simulink model "AttitudeComplementary2"  (Simulink 6.6)
settings: Solver=ode4  StartTime=0.0  StopTime=80  FixedStep=SampleT  RelTol=1e-3
InitFcn:
  | clc
  | Taxi_Var_new
  | failures
  | insInit
  | piccolo_init
values from neighbouring files (symbols this model uses):
  A1 = 0    [Taxi_Var.m]    (also in Taxi_Var_new.m = 0.007)
  Apolar = 0.0899    [Taxi_Var.m]    (also in Taxi_Var_new.m = 0.057)
  APtsamp = 0.005    [failures.m]    (also in piccolo_init.m = 0.05)
  CD0 = 0.0219    [Taxi_Var.m]    (also in Taxi_Var_new.m = 0.022)
  chord = S/span    (= 0.384036716878)    [Taxi_Var.m]    (also in Taxi_Var_new.m = 0.351341681574)
  CL0 = 0.1857    [Taxi_Var.m]    (also in Taxi_Var_new.m = 0.38)
  CLa = 4.6206    [Taxi_Var.m]    (also in Taxi_Var_new.m = 18.5)
  CLa_dot = 1.93    [Taxi_Var.m]    (also in Taxi_Var_new.m = 2.64)
  Clb = -0.0043    [Taxi_Var.m]    (also in Taxi_Var_new.m = -0.06)
  ClDa = 0.1695    [Taxi_Var.m]    (also in Taxi_Var_new.m)
  CLDe = 0.4032    [Taxi_Var.m]    (also in Taxi_Var_new.m = 0.24)
  CLDf = 0.047    [Taxi_Var.m]    (also in Taxi_Var_new.m = 0.4)
  ClDr = 0.0003    [Taxi_Var.m]    (also in Taxi_Var_new.m = 0.055)
  Clp = -0.4425    [Taxi_Var.m]    (also in Taxi_Var_new.m = -0.88)
  CLq = 8.7465    [Taxi_Var.m]    (also in Taxi_Var_new.m = 7.4)
  Clr = 0.0675    [Taxi_Var.m]    (also in Taxi_Var_new.m = 0.04)
  Cm0 = -0.0902    [Taxi_Var.m]    (also in Taxi_Var_new.m = 0.56)
  Cma = -1.3995    [Taxi_Var.m]    (also in Taxi_Var_new.m = -1.58)
  CmDe = -0.9493    [Taxi_Var.m]    (also in Taxi_Var_new.m = -41)
  CmDf = -.021    (= -0.021)    [Taxi_Var.m]    (also in Taxi_Var_new.m)
  Cmq = -10.8760    (= -10.876)    [Taxi_Var.m]    (also in Taxi_Var_new.m = -12)
  Cnb = 0.0281    [Taxi_Var.m]    (also in Taxi_Var_new.m = 0.73)
  CnDa = -0.0031    [Taxi_Var.m]    (also in Taxi_Var_new.m = -0.032)
  CnDr = -0.0882    [Taxi_Var.m]    (also in Taxi_Var_new.m = 0.19)
  Cnp = -0.0695    [Taxi_Var.m]    (also in Taxi_Var_new.m = -0.1)
  Cnr = -0.1045    [Taxi_Var.m]    (also in Taxi_Var_new.m = -0.23)
  CYb = -0.1999    [Taxi_Var.m]    (also in Taxi_Var_new.m = -0.98)
  CYDr = 0.0192    [Taxi_Var.m]    (also in Taxi_Var_new.m = 0.066)
  damax = 25*deg2rad    (= 0.436332312999)    [Taxi_Var.m]    (also in piccolo_init.m)
  damin = -25*deg2rad    (= -0.436332312999)    [Taxi_Var.m]    (also in piccolo_init.m)
  datrim = 0*deg2rad    (= 0)    [Taxi_Var.m]    (also in piccolo_init.m)
  demax = 15*deg2rad    (= 0.261799387799)    [Taxi_Var.m]    (also in piccolo_init.m)
  demin = -15*deg2rad    (= -0.261799387799)    [Taxi_Var.m]    (also in piccolo_init.m)
  detrim = -2.4137*deg2rad    (= -0.0421270121554)    [Taxi_Var.m]    (also in piccolo_init.m = -0.01308996939)
  dfland = 30*deg2rad    (= 0.523598775598)    [Taxi_Var.m]    (also in piccolo_init.m)
  dfmax = 30*deg2rad    (= 0.523598775598)    [Taxi_Var.m]    (also in piccolo_init.m)
  dfmin = 0*deg2rad    (= 0)    [Taxi_Var.m]    (also in piccolo_init.m)
  drmax = 25*deg2rad    (= 0.436332312999)    [Taxi_Var.m]    (also in piccolo_init.m)
  drmin = -25*deg2rad    (= -0.436332312999)    [Taxi_Var.m]    (also in piccolo_init.m)
  drtrim = 0*deg2rad    (= 0)    [Taxi_Var.m]    (also in piccolo_init.m)
  dtmax = 1    [Taxi_Var.m]    (also in piccolo_init.m)
  dtmin = 0    [Taxi_Var.m]    (also in piccolo_init.m)
  dttrim = 0.0725    [Taxi_Var.m]    (also in piccolo_init.m = 0.35)
  Euler_0 = [0; 0; 45]'*pi/180    [Taxi_Var.m]    (also in Taxi_Var_new.m = [0 0 45]'*pi/180)
  heightDown = 0    [insInit.m]
  heightUp = 3000    [insInit.m]
  IdxCmdOrbitRadius = 17    [piccolo_init.m]
  IdxCmdOrbitSense = 18    [piccolo_init.m]
  IdxCmdWp1Alt = 13    [piccolo_init.m]
  IdxCmdWp1Lat = 11    [piccolo_init.m]
  IdxCmdWp1Lon = 12    [piccolo_init.m]
  IdxCmdWp2Alt = 16    [piccolo_init.m]
  IdxCmdWp2Lat = 14    [piccolo_init.m]
  IdxCmdWp2Lon = 15    [piccolo_init.m]
  IdxEstimReserved1 = 4    [piccolo_init.m]
  IdxEstimWEast = 3    [piccolo_init.m]
  IdxEstimWNorth = 2    [piccolo_init.m]
  IdxGainsAltD = 10    [piccolo_init.m]
  IdxGainsAltI = 9    [piccolo_init.m]
  IdxGainsAltP = 8    [piccolo_init.m]
  IdxGainsPdynD = 4    [piccolo_init.m]
  IdxGainsPdynI = 3    [piccolo_init.m]
  IdxGainsPdynP = 2    [piccolo_init.m]
  IdxGainsPitchD = 7    [piccolo_init.m]
  IdxGainsPitchI = 6    [piccolo_init.m]
  IdxGainsPitchP = 5    [piccolo_init.m]
  IdxGainsRollD = 17    [piccolo_init.m]
  IdxGainsRollI = 16    [piccolo_init.m]
  IdxGainsRollP = 15    [piccolo_init.m]
  IdxGainsSlopeElevatorD = 25    [piccolo_init.m]
  IdxGainsSlopeElevatorP = 26    [piccolo_init.m]
  IdxGainsTrackConv = 24    [piccolo_init.m]
  IdxGainsTrackD = 23    [piccolo_init.m]
  IdxGainsTrackI = 22    [piccolo_init.m]
  IdxGainsTrackP = 21    [piccolo_init.m]
  IdxGainsTurnD = 14    [piccolo_init.m]
  IdxGainsTurnI = 13    [piccolo_init.m]
  IdxGainsTurnP = 12    [piccolo_init.m]
  IdxGainsYawD = 20    [piccolo_init.m]
  IdxGainsYawI = 19    [piccolo_init.m]
  IdxGainsYawP = 18    [piccolo_init.m]
  IdxLimitsAileronMax = 11    [piccolo_init.m]
  IdxLimitsAileronMin = 10    [piccolo_init.m]
  IdxLimitsBankMax = 9    [piccolo_init.m]
  IdxLimitsBankMin = 8    [piccolo_init.m]
  IdxLimitsElevatorMax = 13    [piccolo_init.m]
  IdxLimitsElevatorMin = 12    [piccolo_init.m]
  IdxLimitsFlapMax = 19    [piccolo_init.m]
  IdxLimitsFlapMin = 18    [piccolo_init.m]
  IdxLimitsPdynMax = 3    [piccolo_init.m]
  IdxLimitsPdynMin = 2    [piccolo_init.m]
  IdxLimitsRudderMax = 15    [piccolo_init.m]
  IdxLimitsRudderMin = 14    [piccolo_init.m]
  IdxLimitsThrottleMax = 17    [piccolo_init.m]
  IdxLimitsThrottleMin = 16    [piccolo_init.m]
  IdxSensorsAlt = 5    [piccolo_init.m]
  IdxSensorsLat = 3    [piccolo_init.m]
  IdxSensorsLon = 4    [piccolo_init.m]
  IdxSensorsVDown = 8    [piccolo_init.m]
  IdxSensorsVEast = 7    [piccolo_init.m]
  IdxSensorsVNorth = 6    [piccolo_init.m]
  IdxStatesGlobal = 2    [piccolo_init.m]
  IdxStatesManual = 16    [piccolo_init.m]
  IdxStatesMode = 15    [piccolo_init.m]
  ISA_g = 9.815    [Taxi_Var.m]    (also in Taxi_Var_new.m)
  ISA_hmax = 2000    [Taxi_Var.m]    (also in Taxi_Var_new.m)
  ISA_lapse = .0065    (= 0.0065)    [Taxi_Var.m]    (also in Taxi_Var_new.m)
  ISA_P0 = 101325    [Taxi_Var.m]    (also in Taxi_Var_new.m)
  ISA_R = 287    [Taxi_Var.m]    (also in Taxi_Var_new.m)
  ISA_rho0 = 1.225    [Taxi_Var.m]    (also in Taxi_Var_new.m)
  ISA_T0 = 289    [Taxi_Var.m]    (also in Taxi_Var_new.m)
  Ixx = 3.689084    [Taxi_Var.m]    (also in Taxi_Var_new.m = 3.8)
  Iyy = 7.43789    [Taxi_Var.m]    (also in Taxi_Var_new.m = 9.58)
  Izz = 10.22202    [Taxi_Var.m]    (also in Taxi_Var_new.m = 9.68)
  latDown = -100000    [insInit.m]
  latUp = 100000    [insInit.m]
  lonDown = -100000    [insInit.m]
  lonUp = 100000    [insInit.m]
  mass = 22.5    [Taxi_Var.m]    (also in Taxi_Var_new.m = 8.16466266)
  MinThK = 0.075    [Taxi_Var.m]    (also in Taxi_Var_new.m = 0.077)
  ... (+8 more)
undefined symbols (not defined in the file or in its folder): clock, DiscIntNeverNeededParam, Earth, gaind, polesd, WGS84, zerosd
libraries: piccolo_library x60, simulink x51, aerolibconvert2 x14, dspsigops x5, aerolibasang x5, aerolibatmos2 x2, aerolibtransform2 x2, aerolibnav x2, dspmtrx3 x1, aerolibutil x1
(part 2 of 6)

== system AttitudeComplementary2/Accel Comp/get Centripetal ==
  omega : Inport  Orientation=left
  Vb : Inport  Orientation=left  Port=2
  3vector LPF : Subsystem  Orientation=left  mask{flpf=0.1}
      mask prompts: flpf "LowPass Freq"
      mask Display: droots([],-flpf,flpf)
  3x3 Cross Product : aerolibutil/3x3 Cross Product  Orientation=left  SystemSampleTime=-1
  Integer Delay : simulink/Discrete/Integer Delay  Orientation=left  vinit=0.0  samptime=-1  NumDelays=1
  Integer Delay1 : simulink/Discrete/Integer Delay  Orientation=left  vinit=0.0  samptime=-1  NumDelays=1
  Saturation : Saturate  Orientation=left  UpperLimit=10  LowerLimit=-10
  w x Vb : Outport  Orientation=left
  wires:
  Integer Delay1/1 -> 3x3 Cross Product/1
  Integer Delay/1 -> 3x3 Cross Product/2
  omega/1 -> 3vector LPF/1(In1)
  Vb/1 -> Integer Delay/1
  3x3 Cross Product/1 -> Saturation/1  "w x Vb"
  3vector LPF/1(Out1) -> Integer Delay1/1
  Saturation/1 -> w x Vb/1

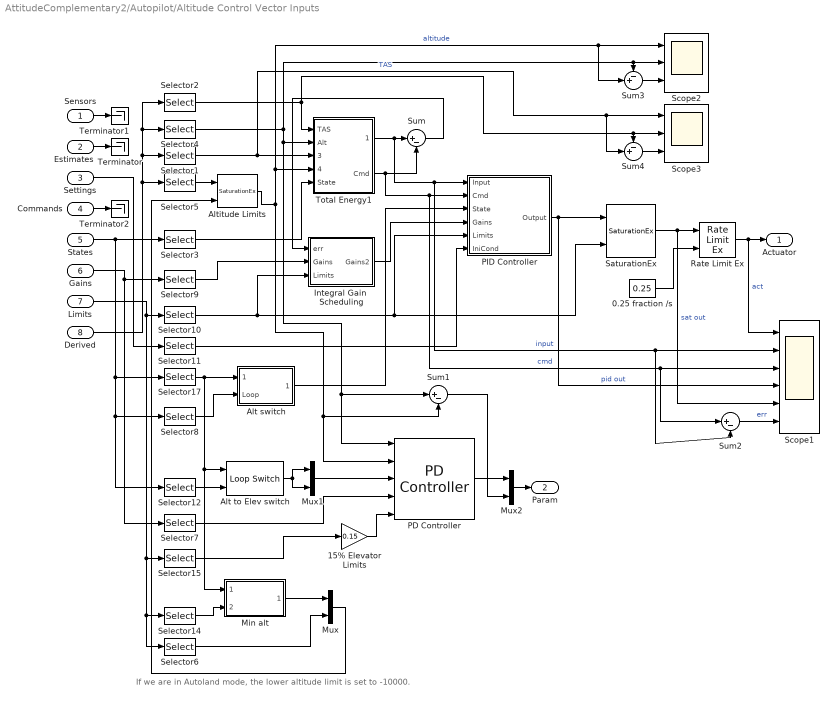
== system AttitudeComplementary2/Autopilot/Altitude Control Vector Inputs ==
  note: If we are in Autoland mode, the lower altitude limit is set to -10000.
  Sensors : Inport  PortDimensions=SizeSensors
  Estimates : Inport  Port=2  PortDimensions=SizeEstim
  Settings : Inport  Port=3  PortDimensions=SizeSet
  Commands : Inport  Port=4  PortDimensions=SizeCmd
  States : Inport  Port=5  PortDimensions=SizeStates
  Gains : Inport  Port=6  PortDimensions=SizeGains
  Limits : Inport  Port=7  PortDimensions=SizeLimits
  Derived : Inport  Port=8  PortDimensions=SizeDrv
  0.25 fraction /s : Constant  Value=0.25
  15% Elevator Limits : Gain  Gain=0.15  SaturateOnIntegerOverflow=on
  Alt switch : Subsystem  AncestorBlock=piccolo_library/Logic/DynP-Alt-Turn switch
  Alt to Elev switch : piccolo_library/Logic/Loop Switch  SystemSampleTime=-1
  Altitude Limits : piccolo_library/Nonlinear/SaturationEx  SystemSampleTime=-1
  Integral Gain  Scheduling : Subsystem
  Min alt : Subsystem
      mask Type: Loop Switch
      mask Description:
      | Select whether this individual loop is enabled or disabled.  This is done based on the specific
      | loop enable state, and the global flag.  In auto or manual steering the loop is on.  In Manual
      | or AutoLaunch the loop should be off.
  Mux : Mux  Inputs=2
  Mux1 : Mux  Inputs=2
  Mux2 : Mux  Inputs=2
  PD Controller : piccolo_library/Controllers/PD Controller  SystemSampleTime=-1  tsamp=tsamp  tdelay=0.5
  PID Controller : Subsystem  AncestorBlock=piccolo_library/Controllers/PID Controller  mask(PID Controller){tsamp=tsamp, tdelay=1}
      mask prompts: tsamp "Sample time:"; tdelay "Time derivative delay:"
      mask help: Generic PID (proportional, integral, derivative) controller with a single input and a single output.
  Rate Limit Ex : piccolo_library/Nonlinear/Rate Limit Ex  SystemSampleTime=-1  T=tsamp
  SaturationEx : piccolo_library/Nonlinear/SaturationEx  SystemSampleTime=-1
  Scope1 : Scope  NumInputPorts=6
      settings: YMin=0.120001~972.462~972.462~0.120001~0.120001~5.25e-006  YMax=0.120001~972.462~972.462~0.120001~0.120001~7e-006
  Scope2 : Scope  NumInputPorts=3
      settings: YMin=855~900.05~-0.475  YMax=945~900.475~-0.05  SaveName=ScopeData14
  Scope3 : Scope  NumInputPorts=3
      settings: YMin=35.0006~35~-0.035  YMax=35.0008~35.035~3.46945e-018  SaveName=ScopeData17
  Selector1 : Selector  IndexOptions=Index vector (dialog)  Indices=IdxDrvTASCmdNom  OutputSizes=1  InputPortWidth=SizeDrv
  Selector10 : Selector  IndexOptions=Index vector (dialog)  Indices=[IdxLimitsThrottleMin IdxLimitsThrottleMax]  OutputSizes=1  InputPortWidth=SizeLimits
  Selector11 : Selector  IndexOptions=Index vector (dialog)  Indices=IdxSetThrottleTrim  OutputSizes=1  InputPortWidth=SizeSet
  Selector12 : Selector  IndexOptions=Index vector (dialog)  Indices=IdxStatesAltToElev  OutputSizes=1  InputPortWidth=SizeStates
  Selector14 : Selector  IndexOptions=Index vector (dialog)  Indices=IdxLimitsAltMin  OutputSizes=1  InputPortWidth=SizeLimits
  Selector15 : Selector  IndexOptions=Index vector (dialog)  Indices=[IdxLimitsElevatorMin IdxLimitsElevatorMax]  OutputSizes=1  InputPortWidth=SizeLimits
  Selector17 : Selector  IndexOptions=Index vector (dialog)  Indices=[IdxStatesGlobal IdxStatesMode IdxStatesManual]  OutputSizes=1  InputPortWidth=SizeStates
  Selector2 : Selector  IndexOptions=Index vector (dialog)  Indices=IdxDrvTAS  OutputSizes=1  InputPortWidth=SizeDrv
  Selector3 : Selector  IndexOptions=Index vector (dialog)  Indices=IdxStatesPdyn  OutputSizes=1  InputPortWidth=SizeStates
  Selector4 : Selector  IndexOptions=Index vector (dialog)  Indices=IdxDrvBaroAlt  OutputSizes=1  InputPortWidth=SizeDrv
  Selector5 : Selector  IndexOptions=Index vector (dialog)  Indices=IdxDrvAltCmd  OutputSizes=1  InputPortWidth=SizeDrv
  Selector6 : Selector  IndexOptions=Index vector (dialog)  Indices=IdxLimitsAltMax  OutputSizes=1  InputPortWidth=SizeLimits
  Selector7 : Selector  IndexOptions=Index vector (dialog)  Indices=[IdxGainsSlopeElevatorP IdxGainsSlopeElevatorD]  OutputSizes=1  InputPortWidth=SizeGains
  Selector8 : Selector  IndexOptions=Index vector (dialog)  Indices=IdxStatesAlt  OutputSizes=1  InputPortWidth=SizeStates
  Selector9 : Selector  IndexOptions=Index vector (dialog)  Indices=[IdxGainsAltP IdxGainsAltI IdxGainsAltD]  OutputSizes=1  InputPortWidth=SizeGains
  Sum : Sum  Inputs=|+-  SaturateOnIntegerOverflow=on
  Sum1 : Sum  Inputs=|+-  SaturateOnIntegerOverflow=on
  Sum2 : Sum  Inputs=|+-  SaturateOnIntegerOverflow=on
  Sum3 : Sum  Inputs=-+|  SaturateOnIntegerOverflow=on
  Sum4 : Sum  Inputs=-+|  SaturateOnIntegerOverflow=on
  Terminator : Terminator
  Terminator1 : Terminator
  Terminator2 : Terminator
  Total Energy1 : Subsystem
      mask Type: Total Energy
      mask Description: Compute the total energy state and command as a sum of kinetic and potential energies, in units of altitude
  Actuator : Outport  OutDataType=fixdt(1,16,0)  OutScaling=[]
  Param : Outport  Port=2  OutDataType=fixdt(1,16,0)  OutScaling=[]
  wires:
  Total Energy1/2(Cmd) -> Sum/2, PID Controller/2(Cmd), Scope1/3, Sum2/1  "cmd"
  Total Energy1/1(Energy) -> Sum/1, PID Controller/1(Input), Scope1/2, Sum2/2  "input"
  Selector3/1 -> Total Energy1/5(State)
  Selector1/1 -> Total Energy1/3(TASCmd), Scope3/1, Sum4/2  "TAS"
  PD Controller/1 -> Mux2/1
  Mux2/1 -> Param/1
  Sum1/1 -> Mux2/2
  Commands/1 -> Terminator2/1
  States/1 -> Selector3/1, Selector12/1, Selector8/1, Selector17/1
  Sum/1 -> Integral Gain  Scheduling/1(err)
  Selector7/1 -> PD Controller/4
  Mux1/1 -> PD Controller/3
  Alt to Elev switch/1 -> Mux1/2, Mux1/1
  Selector15/1 -> 15% Elevator Limits/1
  15% Elevator Limits/1 -> PD Controller/5
  Selector9/1 -> Integral Gain  Scheduling/2(Gains)
  Integral Gain  Scheduling/1(Gains2) -> PID Controller/4(Gains)
  Mux/1 -> Altitude Limits/2
  Selector6/1 -> Mux/2
  Min alt/1(MinAltOut) -> Mux/1
  Selector14/1 -> Min alt/2(MinAlt)
  Selector12/1 -> Alt to Elev switch/2
  PID Controller/1(Output) -> SaturationEx/1, Scope1/4  "pid out"
  Derived/1 -> Selector1/1, Selector4/1, Selector2/1, Selector5/1
  Selector5/1 -> Altitude Limits/1
  Altitude Limits/1 -> Sum1/2, PD Controller/2, Total Energy1/4(AltCmd), Scope2/1, Sum3/2  "altitude"
  Selector4/1 -> Total Energy1/2(Alt), Sum1/1, PD Controller/1, Scope2/2, Sum3/1
  Selector2/1 -> Total Energy1/1(TAS), Scope3/2, Sum4/1
  Sensors/1 -> Terminator1/1
  Rate Limit Ex/1 -> Actuator/1, Scope1/1  "act"
  0.25 fraction /s/1 -> Rate Limit Ex/2
  SaturationEx/1 -> Rate Limit Ex/1, Scope1/5  "sat out"
  Selector10/1 -> Integral Gain  Scheduling/3(Limits), SaturationEx/2, PID Controller/5(Limits)
  Limits/1 -> Selector15/1, Selector6/1, Selector14/1, Selector10/1
  Gains/1 -> Selector7/1, Selector9/1
  Selector11/1 -> PID Controller/6(IniCond)
  Settings/1 -> Selector11/1
  Selector17/1 -> Alt switch/1(Globals), Min alt/1(Globals), Alt to Elev switch/1
  Selector8/1 -> Alt switch/2(Loop)
  Alt switch/1(TriOut) -> PID Controller/3(State)
  Estimates/1 -> Terminator/1
  Sum2/1 -> Scope1/6  "err"
  Sum3/1 -> Scope2/3
  Sum4/1 -> Scope3/3

== system AttitudeComplementary2/Autopilot/Flap Control Vector Inputs ==
  Sensors : Inport  PortDimensions=SizeSensors
  Estimates : Inport  Port=2  PortDimensions=SizeEstim
  Settings : Inport  Port=3  PortDimensions=SizeSet
  Commands : Inport  Port=4  PortDimensions=SizeCmd
  States : Inport  Port=5  PortDimensions=SizeStates
  Gains : Inport  Port=6  PortDimensions=SizeGains
  Limits : Inport  Port=7  PortDimensions=SizeLimits
  Derived : Inport  Port=8  PortDimensions=SizeDrv
  5 deg/s : Constant  Value=10*pi/180
  Direct Flap Control : Selector  IndexOptions=Index vector (dialog)  Indices=IdxCmdFlap  OutputSizes=1  InputPortWidth=SizeCmd
  Flap Loop Switch : piccolo_library/Logic/Loop Switch  SystemSampleTime=-1
  Landing Flap : Selector  IndexOptions=Index vector (dialog)  Indices=IdxSetLandingFlap  OutputSizes=1  InputPortWidth=SizeSet
  Rate Limit Ex : piccolo_library/Nonlinear/Rate Limit Ex  SystemSampleTime=-1  T=tsamp
  SaturationEx : piccolo_library/Nonlinear/SaturationEx  SystemSampleTime=-1
  Selector1 : Selector  IndexOptions=Index vector (dialog)  Indices=[IdxStatesGlobal IdxStatesMode IdxStatesManual]  OutputSizes=1  InputPortWidth=SizeStates
  Selector10 : Selector  IndexOptions=Index vector (dialog)  Indices=[IdxLimitsFlapMin IdxLimitsFlapMax]  OutputSizes=1  InputPortWidth=SizeLimits
  Selector12 : Selector  IndexOptions=Index vector (dialog)  Indices=IdxStatesSlope  OutputSizes=1  InputPortWidth=SizeStates
  Selector2 : Selector  IndexOptions=Index vector (dialog)  Indices=IdxStatesFlap  OutputSizes=1  InputPortWidth=SizeStates
  Switch : Switch  Threshold=0.5  SaturateOnIntegerOverflow=on
  Switch1 : Switch  Threshold=0.5  SaturateOnIntegerOverflow=on
  Terminator{1..4} (4 alike) : Terminator
  Zero : Constant  Value=0
  Actuator : Outport  OutDataType=fixdt(1,16,0)  OutScaling=[]
  wires:
  Sensors/1 -> Terminator1/1
  Selector10/1 -> SaturationEx/2
  Selector12/1 -> Switch/2
  Direct Flap Control/1 -> Switch/3
  Landing Flap/1 -> Switch/1
  Estimates/1 -> Terminator2/1
  Gains/1 -> Terminator3/1
  Derived/1 -> Terminator4/1
  Settings/1 -> Landing Flap/1
  Commands/1 -> Direct Flap Control/1
  States/1 -> Selector12/1, Selector2/1, Selector1/1
  Limits/1 -> Selector10/1
  Switch/1 -> Switch1/1
  Flap Loop Switch/1 -> Switch1/2
  Switch1/1 -> SaturationEx/1
  Selector1/1 -> Flap Loop Switch/1
  Selector2/1 -> Flap Loop Switch/2
  Zero/1 -> Switch1/3
  SaturationEx/1 -> Rate Limit Ex/1
  Rate Limit Ex/1 -> Actuator/1
  5 deg/s/1 -> Rate Limit Ex/2

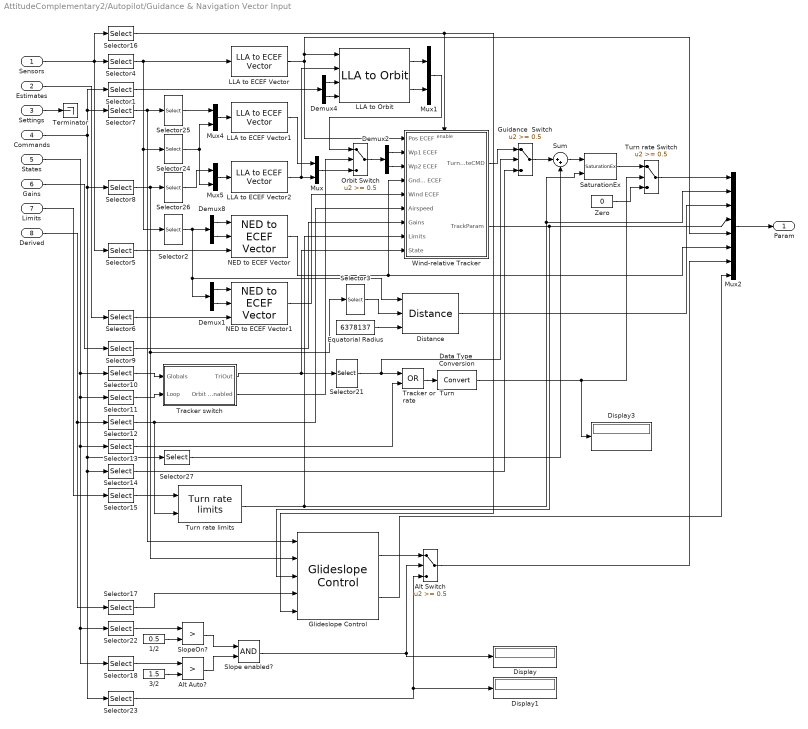
== system AttitudeComplementary2/Autopilot/Guidance & Navigation Vector Input ==
  Sensors : Inport  PortDimensions=SizeSensors
  Estimates : Inport  Port=2  PortDimensions=SizeEstim
  Settings : Inport  Port=3  PortDimensions=SizeSet
  Commands : Inport  Port=4  PortDimensions=SizeCmd
  States : Inport  Port=5  PortDimensions=SizeStates
  Gains : Inport  Port=6  PortDimensions=SizeGains
  Limits : Inport  Port=7  PortDimensions=SizeLimits
  Derived : Inport  Port=8  PortDimensions=SizeDrv
  1/2 : Constant  Value=0.5
  3/2 : Constant  Value=1.5
  Alt Auto? : RelationalOperator  Operator=>
  Alt Switch : Switch  Threshold=0.5  SaturateOnIntegerOverflow=on
  Data Type  Conversion : DataTypeConversion  OutDataTypeMode=double  OutDataType=fixdt(1,16,0)  OutScaling=[]  SaturateOnIntegerOverflow=on  RndMeth=Zero
  Demux{1..2,4,8} (4 alike) : Demux  Outputs=2
  Display : Display
  Display1 : Display
  Display3 : Display
  Distance : piccolo_library/Transformations/Distance  SystemSampleTime=-1
  Equatorial Radius : Constant  Value=6378137
  Glideslope Control : piccolo_library/Controllers/Guidance/Glideslope Control  SystemSampleTime=-1  tsamp=tsamp  aptsamp=aptsamp
  Guidance  Switch : Switch  Threshold=0.5  SaturateOnIntegerOverflow=on
  LLA to ECEF Vector : piccolo_library/Transformations/LLA to ECEF Vector  SystemSampleTime=-1
  LLA to ECEF Vector1 : piccolo_library/Transformations/LLA to ECEF Vector  SystemSampleTime=-1
  LLA to ECEF Vector2 : piccolo_library/Transformations/LLA to ECEF Vector  SystemSampleTime=-1
  LLA to Orbit : piccolo_library/Controllers/Guidance/LLA to Orbit  SystemSampleTime=-1
  Mux{,1,4..5} (4 alike) : Mux  Inputs=2
  Mux2 : Mux  Inputs=[1 2 1 5 3 3 1 3]
  NED to ECEF Vector : piccolo_library/Transformations/NED to ECEF Vector  SystemSampleTime=-1
  NED to ECEF Vector1 : piccolo_library/Transformations/NED to ECEF Vector  SystemSampleTime=-1
  Orbit Switch : Switch  Threshold=0.5  SaturateOnIntegerOverflow=on
  SaturationEx : piccolo_library/Nonlinear/SaturationEx  SystemSampleTime=-1
  Selector1 : Selector  IndexOptions=Index vector (dialog)  Indices=[IdxCmdOrbitRadius IdxCmdOrbitSense]  OutputSizes=1  InputPortWidth=SizeCmd
  Selector10 : Selector  IndexOptions=Index vector (dialog)  Indices=[IdxStatesGlobal IdxStatesMode IdxStatesManual]  OutputSizes=1  InputPortWidth=SizeStates
  Selector11 : Selector  IndexOptions=Index vector (dialog)  Indices=IdxStatesTracker  OutputSizes=1  InputPortWidth=SizeStates
  Selector12 : Selector  IndexOptions=Index vector (dialog)  Indices=IdxDrvTAS  OutputSizes=1  InputPortWidth=SizeDrv
  Selector13 : Selector  IndexOptions=Index vector (dialog)  Indices=IdxStatesTurnRate  OutputSizes=1  InputPortWidth=SizeStates
  Selector14 : Selector  IndexOptions=Index vector (dialog)  Indices=IdxCmdTurnRate  OutputSizes=1  InputPortWidth=SizeCmd
  Selector15 : Selector  IndexOptions=Index vector (dialog)  Indices=[IdxLimitsBankMin IdxLimitsBankMax]  OutputSizes=1  InputPortWidth=SizeLimits
  Selector16 : Selector  IndexOptions=Index vector (dialog)  Indices=IdxSensorsGPSNew  OutputSizes=1  InputPortWidth=SizeSensors
  Selector17 : Selector  IndexOptions=Index vector (dialog)  Indices=IdxDrvBaroAlt  OutputSizes=1  InputPortWidth=SizeDrv
  Selector18 : Selector  IndexOptions=Index vector (dialog)  Indices=IdxStatesAlt  OutputSizes=1  InputPortWidth=SizeStates
  Selector{2..3,25..26} (4 alike) : Selector  IndexOptions=Index vector (dialog)  Indices=[1 2]  OutputSizes=1  InputPortWidth=3
  Selector21 : Selector  IndexOptions=Index vector (dialog)  Indices=2  OutputSizes=1  InputPortWidth=3
  Selector22 : Selector  IndexOptions=Index vector (dialog)  Indices=IdxStatesSlope  OutputSizes=1  InputPortWidth=SizeStates
  Selector23 : Selector  IndexOptions=Index vector (dialog)  Indices=IdxCmdAlt  OutputSizes=1  InputPortWidth=SizeCmd
  Selector24 : Selector  IndexOptions=Index vector (dialog)  Indices=3  OutputSizes=1  InputPortWidth=3
  Selector27 : Selector  IndexOptions=Index vector (dialog)  Indices=IdxCmdTurnRateShift  OutputSizes=1  InputPortWidth=SizeCmd
  Selector4 : Selector  IndexOptions=Index vector (dialog)  Indices=[IdxSensorsLat IdxSensorsLon IdxSensorsAlt]  OutputSizes=1  InputPortWidth=SizeSensors
  Selector5 : Selector  IndexOptions=Index vector (dialog)  Indices=[IdxSensorsVNorth IdxSensorsVEast IdxSensorsVDown]  OutputSizes=1  InputPortWidth=SizeSensors
  Selector6 : Selector  IndexOptions=Index vector (dialog)  Indices=[IdxEstimWNorth IdxEstimWEast IdxEstimReserved1]  OutputSizes=1  InputPortWidth=SizeEstim
  Selector7 : Selector  IndexOptions=Index vector (dialog)  Indices=[IdxCmdWp1Lat IdxCmdWp1Lon IdxCmdWp1Alt]  OutputSizes=1  InputPortWidth=SizeCmd
  Selector8 : Selector  IndexOptions=Index vector (dialog)  Indices=[IdxCmdWp2Lat IdxCmdWp2Lon IdxCmdWp2Alt]  OutputSizes=1  InputPortWidth=SizeCmd
  Selector9 : Selector  IndexOptions=Index vector (dialog)  Indices=[IdxGainsTrackP IdxGainsTrackI IdxGainsTrackD IdxGainsTrackConv]  OutputSizes=1  InputPortWidth=SizeGains
  Slope enabled? : Logic  AllPortsSameDT=off
  SlopeOn? : RelationalOperator  Operator=>
  Sum : Sum  Inputs=|++  SaturateOnIntegerOverflow=on
  Terminator : Terminator
  Tracker or  Turn rate : Logic  Operator=OR  AllPortsSameDT=off
  Tracker switch : Subsystem  AncestorBlock=piccolo_library/Logic/Tracker switch
  Turn rate Switch : Switch  Threshold=0.5  SaturateOnIntegerOverflow=on
  Turn rate limits : piccolo_library/Flight Mechanics/Turn rate limits  SystemSampleTime=-1
  Wind-relative Tracker : Subsystem  AncestorBlock=piccolo_library/Controllers/Guidance/Wind-relative Tracker  mask(Wind-relative Tracker){tsamp=tsamp}
      mask prompts: tsamp "Sample time:"
      mask help: A lateral track control law that takes into account the wind speed.
  Zero : Constant  Value=0
  Param : Outport  OutDataType=fixdt(1,16,0)  OutScaling=[]
  wires:
  Slope enabled?/1 -> Alt Switch/2, Display/1
  Alt Auto?/1 -> Slope enabled?/2
  SlopeOn?/1 -> Slope enabled?/1
  3/2/1 -> Alt Auto?/2
  Selector18/1 -> Alt Auto?/1
  Selector22/1 -> SlopeOn?/1
  1/2/1 -> SlopeOn?/2
  Selector21/1 -> Tracker or  Turn rate/1, Guidance  Switch/2
  Selector27/1 -> Sum/2
  Sum/1 -> SaturationEx/1
  Guidance  Switch/1 -> Sum/1
  Glideslope Control/2 -> Mux2/8
  Glideslope Control/1 -> Alt Switch/1
  Selector17/1 -> Glideslope Control/4
  Selector26/1 -> Mux5/1
  Selector7/1 -> Glideslope Control/1, Selector25/1
  Selector25/1 -> Mux4/1
  Selector24/1 -> Mux5/2, Mux4/2
  Mux5/1 -> LLA to ECEF Vector2/1
  Mux4/1 -> LLA to ECEF Vector1/1
  Alt Switch/1 -> Mux2/7
  Selector23/1 -> Alt Switch/3, Display1/1
  LLA to Orbit/2 -> Mux1/2
  LLA to Orbit/1 -> Mux1/1
  Selector1/1 -> Demux4/1
  Demux4/2 -> LLA to Orbit/4
  Demux4/1 -> LLA to Orbit/3
  Selector16/1 -> Glideslope Control/5, Wind-relative Tracker/Enable
  Settings/1 -> Terminator/1
  Data Type  Conversion/1 -> Turn rate Switch/2, Display3/1
  Wind-relative Tracker/2(TrackParam) -> Glideslope Control/3, Mux2/4
  Distance/1 -> Mux2/3
  Zero/1 -> Turn rate Switch/3
  SaturationEx/1 -> Turn rate Switch/1
  Tracker or  Turn rate/1 -> Data Type  Conversion/1
  Selector13/1 -> Tracker or  Turn rate/2
  Turn rate limits/1 -> Mux2/2, SaturationEx/2, Wind-relative Tracker/8(Limits)
  Limits/1 -> Selector15/1
  Selector15/1 -> Turn rate limits/1
  Selector14/1 -> Guidance  Switch/3
  Wind-relative Tracker/1(TurnRateCMD) -> Guidance  Switch/1
  Mux2/1 -> Param/1
  Tracker switch/1(TriOut) -> Wind-relative Tracker/9(State), Selector21/1
  Tracker switch/2(Orbit Enabled) -> Orbit Switch/2
  Selector11/1 -> Tracker switch/2(Loop)
  Selector10/1 -> Tracker switch/1(Globals)
  Derived/1 -> Selector17/1, Selector12/1
  States/1 -> Selector18/1, Selector22/1, Selector13/1, Selector11/1, Selector10/1
  Gains/1 -> Selector9/1
  Commands/1 -> Selector1/1, Selector7/1, Selector27/1, Selector23/1, Selector14/1, Selector8/1
  Selector8/1 -> Glideslope Control/2, Selector3/1, Selector26/1
  Estimates/1 -> Selector6/1
  Selector5/1 -> NED to ECEF Vector/3
  Sensors/1 -> Selector16/1, Selector5/1, Selector4/1
  Selector4/1 -> Selector2/1, Selector24/1, LLA to ECEF Vector/1
  Demux8/1 -> NED to ECEF Vector/1
  Demux8/2 -> NED to ECEF Vector/2
  Selector2/1 -> Demux8/1, Demux1/1, Distance/1
  Demux1/1 -> NED to ECEF Vector1/1
  Demux1/2 -> NED to ECEF Vector1/2
  Selector6/1 -> NED to ECEF Vector1/3
  LLA to ECEF Vector/1 -> LLA to Orbit/1, Mux2/5, Wind-relative Tracker/1(Pos ECEF)
  LLA to ECEF Vector2/1 -> LLA to Orbit/2, Mux/2
  Selector9/1 -> Wind-relative Tracker/7(Gains)
  LLA to ECEF Vector1/1 -> Mux/1
  Mux/1 -> Orbit Switch/3
  Mux1/1 -> Orbit Switch/1
  Demux2/1 -> Wind-relative Tracker/2(Wp1 ECEF)
  Demux2/2 -> Wind-relative Tracker/3(Wp2 ECEF)
  Orbit Switch/1 -> Demux2/1
  NED to ECEF Vector/1 -> Mux2/6, Wind-relative Tracker/4(Gndspd ECEF)
  NED to ECEF Vector1/1 -> Wind-relative Tracker/5(Wind ECEF)
  Selector12/1 -> Turn rate limits/2, Wind-relative Tracker/6(Airspeed)
  Equatorial Radius/1 -> Distance/3
  Selector3/1 -> Distance/2
  Turn rate Switch/1 -> Mux2/1

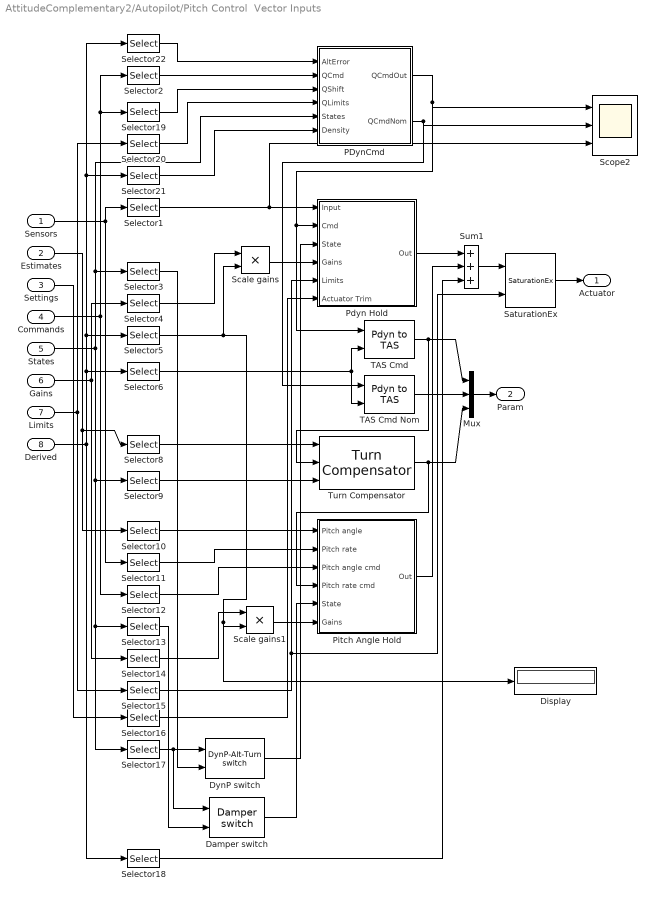
== system AttitudeComplementary2/Autopilot/Pitch Control  Vector Inputs ==
  Sensors : Inport  PortDimensions=SizeSensors
  Estimates : Inport  Port=2  PortDimensions=SizeEstim
  Settings : Inport  Port=3  PortDimensions=SizeSet
  Commands : Inport  Port=4  PortDimensions=SizeCmd
  States : Inport  Port=5  PortDimensions=SizeStates
  Gains : Inport  Port=6  PortDimensions=SizeGains
  Limits : Inport  Port=7  PortDimensions=SizeLimits
  Derived : Inport  Port=8  PortDimensions=SizeDrv
  Damper switch : piccolo_library/Logic/Damper switch  SystemSampleTime=-1
  Display : Display
  DynP switch : piccolo_library/Logic/DynP-Alt-Turn switch  SystemSampleTime=-1
  Mux : Mux  Inputs=3
  PDynCmd : Subsystem
  Pdyn Hold : Subsystem  AncestorBlock=piccolo_library/Controllers/Longitudinal/Pdyn Hold  mask(Dynamic pressure hold){tsamp=tsamp}
      mask prompts: tsamp "Sample time:"
      mask help: Control the dynamic pressure using elevator command.
  Pitch Angle Hold : Subsystem  AncestorBlock=piccolo_library/Controllers/Longitudinal/Pitch Angle Hold  mask(Pitch angle hold){tsamp=tsamp}
      mask prompts: tsamp "Sample time:"
      mask help: Pitch angle hold with proportional and derivative terms.
  SaturationEx : piccolo_library/Nonlinear/SaturationEx  SystemSampleTime=-1
  Scale gains : Product  SaturateOnIntegerOverflow=on  InputSameDT=on
  Scale gains1 : Product  SaturateOnIntegerOverflow=on  InputSameDT=on
  Scope2 : Scope  NumInputPorts=3
      settings: YMin=687.696~687.696~688.4  YMax=687.696~687.696~688.775  SaveName=ScopeData3
  Selector1 : Selector  IndexOptions=Index vector (dialog)  Indices=IdxSensorsPdyn  OutputSizes=1  InputPortWidth=SizeSensors
  Selector10 : Selector  IndexOptions=Index vector (dialog)  Indices=IdxEstimPitchAngle  OutputSizes=1  InputPortWidth=SizeEstim
  Selector11 : Selector  IndexOptions=Index vector (dialog)  Indices=IdxSensorsPitchRate  OutputSizes=1  InputPortWidth=SizeSensors
  Selector12 : Selector  IndexOptions=Index vector (dialog)  Indices=IdxCmdPitchAngle  OutputSizes=1  InputPortWidth=SizeCmd
  Selector13 : Selector  IndexOptions=Index vector (dialog)  Indices=IdxStatesPitch  OutputSizes=1  InputPortWidth=SizeStates
  Selector14 : Selector  IndexOptions=Index vector (dialog)  Indices=[IdxGainsPitchP IdxGainsPitchI IdxGainsPitchD]  OutputSizes=1  InputPortWidth=SizeGains
  Selector15 : Selector  IndexOptions=Index vector (dialog)  Indices=[IdxLimitsElevatorMin IdxLimitsElevatorMax]  OutputSizes=1  InputPortWidth=SizeLimits
  Selector16 : Selector  IndexOptions=Index vector (dialog)  Indices=IdxSetElevatorTrim  OutputSizes=1  InputPortWidth=SizeSet
  Selector17 : Selector  IndexOptions=Index vector (dialog)  Indices=[IdxStatesGlobal IdxStatesMode IdxStatesManual]  OutputSizes=1  InputPortWidth=SizeStates
  Selector18 : Selector  IndexOptions=Index vector (dialog)  Indices=IdxDrvSlopeElevator  OutputSizes=1  InputPortWidth=SizeDrv
  Selector19 : Selector  IndexOptions=Index vector (dialog)  Indices=IdxCmdPdynShift  OutputSizes=1  InputPortWidth=SizeCmd
  Selector2 : Selector  IndexOptions=Index vector (dialog)  Indices=IdxCmdPdyn  OutputSizes=1  InputPortWidth=SizeCmd
  Selector20 : Selector  IndexOptions=Index vector (dialog)  Indices=[IdxLimitsPdynMin IdxLimitsPdynMax]  OutputSizes=1  InputPortWidth=SizeLimits
  Selector21 : Selector  IndexOptions=Index vector (dialog)  Indices=IdxDrvDensity  OutputSizes=1  InputPortWidth=SizeDrv
  Selector22 : Selector  IndexOptions=Index vector (dialog)  Indices=IdxDrvAltError  OutputSizes=1  InputPortWidth=SizeDrv
  Selector3 : Selector  IndexOptions=Index vector (dialog)  Indices=IdxStatesPdyn  OutputSizes=1  InputPortWidth=SizeStates
  Selector4 : Selector  IndexOptions=Index vector (dialog)  Indices=[IdxGainsPdynP IdxGainsPdynI IdxGainsPdynD]  OutputSizes=1  InputPortWidth=SizeGains
  Selector5 : Selector  IndexOptions=Index vector (dialog)  Indices=IdxDrvGainScaler  OutputSizes=1  InputPortWidth=SizeDrv
  Selector6 : Selector  IndexOptions=Index vector (dialog)  Indices=IdxDrvDensity  OutputSizes=1  InputPortWidth=SizeDrv
  Selector8 : Selector  IndexOptions=Index vector (dialog)  Indices=IdxEstimRollAngle  OutputSizes=1  InputPortWidth=SizeEstim
  Selector9 : Selector  IndexOptions=Index vector (dialog)  Indices=IdxStatesTurnComp  OutputSizes=1  InputPortWidth=SizeStates
  Sum1 : Sum  Inputs=+++  SaturateOnIntegerOverflow=on  InputSameDT=on
  TAS Cmd : piccolo_library/Flight Mechanics/Pdyn to TAS  SystemSampleTime=-1
  TAS Cmd Nom : piccolo_library/Flight Mechanics/Pdyn to TAS  SystemSampleTime=-1
  Turn Compensator : piccolo_library/Controllers/Longitudinal/Turn Compensator  SystemSampleTime=-1
  Actuator : Outport  OutDataType=fixdt(1,16,0)  OutScaling=[]
  Param : Outport  Port=2  OutDataType=fixdt(1,16,0)  OutScaling=[]
  wires:
  PDynCmd/2(QCmdNom) -> TAS Cmd Nom/1, Scope2/2
  TAS Cmd Nom/1 -> Mux/2
  PDynCmd/1(QCmdOut) -> TAS Cmd/1, Pdyn Hold/2(Cmd), Scope2/1
  Selector22/1 -> PDynCmd/1(AltError)
  Selector21/1 -> PDynCmd/6(Density)
  Selector20/1 -> PDynCmd/4(QLimits)
  Selector19/1 -> PDynCmd/3(QShift)
  Selector2/1 -> PDynCmd/2(QCmd)
  Damper switch/1 -> Pitch Angle Hold/5(State)
  DynP switch/1 -> Pdyn Hold/3(State)
  Selector9/1 -> Turn Compensator/3
  Selector18/1 -> Sum1/3
  Selector13/1 -> Damper switch/2
  Selector3/1 -> DynP switch/2
  Selector17/1 -> Damper switch/1, DynP switch/1
  Mux/1 -> Param/1
  Settings/1 -> Selector16/1
  Selector16/1 -> Pdyn Hold/6(Actuator Trim)
  Estimates/1 -> Selector8/1, Selector10/1
  Limits/1 -> Selector20/1, Selector15/1
  Derived/1 -> Selector18/1, Selector22/1, Selector21/1, Selector5/1, Selector6/1
  Gains/1 -> Selector14/1, Selector4/1
  States/1 -> PDynCmd/5(States), Selector3/1, Selector17/1, Selector13/1, Selector9/1
  Commands/1 -> Selector19/1, Selector2/1, Selector12/1
  Sensors/1 -> Selector11/1, Selector1/1
  Selector1/1 -> Pdyn Hold/1(Input), Scope2/3
  TAS Cmd/1 -> Mux/1, Turn Compensator/2
  Selector8/1 -> Turn Compensator/1
  Selector10/1 -> Pitch Angle Hold/1(Pitch angle)
  Selector11/1 -> Pitch Angle Hold/2(Pitch rate)
  Turn Compensator/1 -> Mux/3, Pitch Angle Hold/4(Pitch rate cmd)
  Selector12/1 -> Pitch Angle Hold/3(Pitch angle cmd)
  Scale gains/1 -> Pdyn Hold/4(Gains)
  Selector4/1 -> Scale gains/1
  Selector5/1 -> Scale gains/2, Scale gains1/2, Display/1
  Selector6/1 -> TAS Cmd Nom/2, TAS Cmd/2
  Scale gains1/1 -> Pitch Angle Hold/6(Gains)
  Selector14/1 -> Scale gains1/1
  Selector15/1 -> Pdyn Hold/5(Limits), SaturationEx/2
  Pdyn Hold/1(Out) -> Sum1/1
  Pitch Angle Hold/1(Out) -> Sum1/2
  Sum1/1 -> SaturationEx/1
  SaturationEx/1 -> Actuator/1

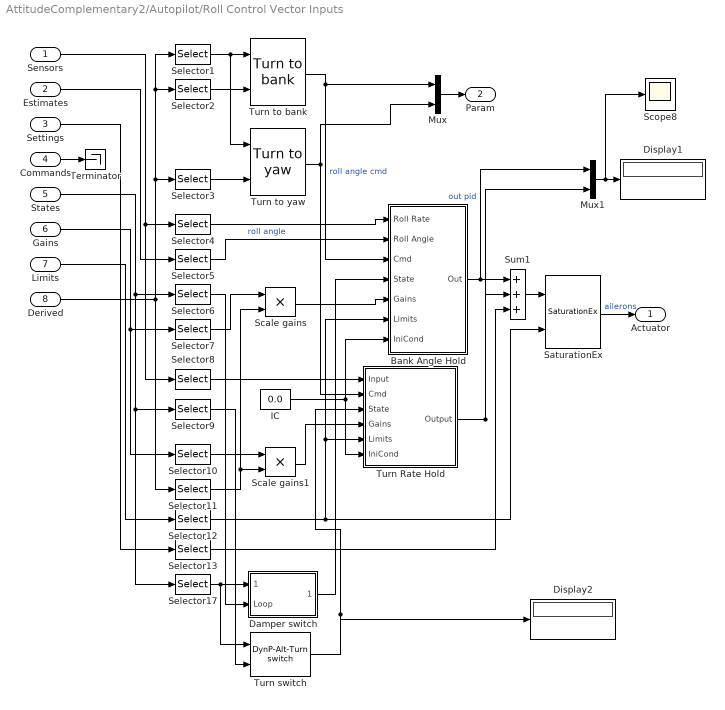
== system AttitudeComplementary2/Autopilot/Roll Control Vector Inputs ==
  Sensors : Inport  PortDimensions=SizeSensors
  Estimates : Inport  Port=2  PortDimensions=SizeEstim
  Settings : Inport  Port=3  PortDimensions=SizeSet
  Commands : Inport  Port=4  PortDimensions=SizeCmd
  States : Inport  Port=5  PortDimensions=SizeStates
  Gains : Inport  Port=6  PortDimensions=SizeGains
  Limits : Inport  Port=7  PortDimensions=SizeLimits
  Derived : Inport  Port=8  PortDimensions=SizeDrv
  Bank Angle Hold : Subsystem  AncestorBlock=piccolo_library/Controllers/Lateral/Bank Angle Hold
  Damper switch : Subsystem  AncestorBlock=piccolo_library/Logic/Damper switch
  Display1 : Display
  Display2 : Display
  IC : Constant  Value=0.0
  Mux : Mux  Inputs=2
  Mux1 : Mux  Inputs=2
  SaturationEx : piccolo_library/Nonlinear/SaturationEx  SystemSampleTime=-1
  Scale gains : Product  SaturateOnIntegerOverflow=on  InputSameDT=on
  Scale gains1 : Product  SaturateOnIntegerOverflow=on  InputSameDT=on
  Scope8 : Scope
      settings: YMin=-0.6  YMax=0.6  SaveName=ScopeData26
  Selector1 : Selector  IndexOptions=Index vector (dialog)  Indices=IdxDrvTurnRateCmd  OutputSizes=1  InputPortWidth=SizeDrv
  Selector10 : Selector  IndexOptions=Index vector (dialog)  Indices=[IdxGainsTurnP IdxGainsTurnI IdxGainsTurnD]  OutputSizes=1  InputPortWidth=SizeGains
  Selector11 : Selector  IndexOptions=Index vector (dialog)  Indices=IdxDrvGainScaler  OutputSizes=1  InputPortWidth=SizeDrv
  Selector12 : Selector  IndexOptions=Index vector (dialog)  Indices=[IdxLimitsAileronMin IdxLimitsAileronMax]  OutputSizes=1  InputPortWidth=SizeLimits
  Selector13 : Selector  IndexOptions=Index vector (dialog)  Indices=IdxSetAileronTrim  OutputSizes=1  InputPortWidth=SizeSet
  Selector17 : Selector  IndexOptions=Index vector (dialog)  Indices=[IdxStatesGlobal IdxStatesMode IdxStatesManual]  OutputSizes=1  InputPortWidth=SizeStates
  Selector2 : Selector  IndexOptions=Index vector (dialog)  Indices=IdxDrvTAS  OutputSizes=1  InputPortWidth=SizeDrv
  Selector3 : Selector  IndexOptions=Index vector (dialog)  Indices=IdxDrvTAS  OutputSizes=1  InputPortWidth=SizeDrv
  Selector4 : Selector  IndexOptions=Index vector (dialog)  Indices=IdxSensorsRollRate  OutputSizes=1  InputPortWidth=SizeSensors
  Selector5 : Selector  IndexOptions=Index vector (dialog)  Indices=IdxEstimRollAngle  OutputSizes=1  InputPortWidth=SizeEstim
  Selector6 : Selector  IndexOptions=Index vector (dialog)  Indices=IdxStatesRoll  OutputSizes=1  InputPortWidth=SizeStates
  Selector7 : Selector  IndexOptions=Index vector (dialog)  Indices=[IdxGainsRollP IdxGainsRollI IdxGainsRollD]  OutputSizes=1  InputPortWidth=SizeGains
  Selector8 : Selector  IndexOptions=Index vector (dialog)  Indices=IdxSensorsYawRate  OutputSizes=1  InputPortWidth=SizeSensors
  Selector9 : Selector  IndexOptions=Index vector (dialog)  Indices=IdxStatesTurnRate  OutputSizes=1  InputPortWidth=SizeStates
  Sum1 : Sum  Inputs=+++  SaturateOnIntegerOverflow=on  InputSameDT=on
  Terminator : Terminator
  Turn Rate Hold : Subsystem  AncestorBlock=piccolo_library/Controllers/PID Controller  mask(PID Controller){tsamp=tsamp, tdelay=0.25}
      mask prompts: tsamp "Sample time:"; tdelay "Time derivative delay:"
      mask help: Generic PID (proportional, integral, derivative) controller with a single input and a single output.
  Turn switch : piccolo_library/Logic/DynP-Alt-Turn switch  SystemSampleTime=-1
  Turn to bank : piccolo_library/Flight Mechanics/Turn to bank  SystemSampleTime=-1
  Turn to yaw : piccolo_library/Flight Mechanics/Turn to yaw  SystemSampleTime=-1
  Actuator : Outport  OutDataType=fixdt(1,16,0)  OutScaling=[]
  Param : Outport  Port=2  OutDataType=fixdt(1,16,0)  OutScaling=[]
  wires:
  IC/1 -> Turn Rate Hold/6(IniCond), Bank Angle Hold/7(IniCond)
  Commands/1 -> Terminator/1
  Turn switch/1 -> Turn Rate Hold/3(State), Display2/1
  Selector9/1 -> Turn switch/2
  Damper switch/1(TriOut) -> Bank Angle Hold/4(State)
  Selector6/1 -> Damper switch/2(Loop)
  Selector17/1 -> Damper switch/1(Globals), Turn switch/1
  Mux/1 -> Param/1
  Settings/1 -> Selector13/1
  Selector13/1 -> Sum1/3
  Limits/1 -> Selector12/1
  Gains/1 -> Selector10/1, Selector7/1
  States/1 -> Selector17/1, Selector9/1, Selector6/1
  Estimates/1 -> Selector5/1
  Sensors/1 -> Selector8/1, Selector4/1
  Derived/1 -> Selector11/1, Selector1/1, Selector2/1, Selector3/1
  SaturationEx/1 -> Actuator/1  "ailerons"
  Sum1/1 -> SaturationEx/1
  Turn Rate Hold/1(Output) -> Sum1/2, Mux1/2
  Bank Angle Hold/1(Out) -> Sum1/1, Mux1/1  "out pid"
  Selector12/1 -> SaturationEx/2, Turn Rate Hold/5(Limits), Bank Angle Hold/6(Limits)
  Selector11/1 -> Scale gains1/2, Scale gains/2
  Selector10/1 -> Scale gains1/1
  Scale gains1/1 -> Turn Rate Hold/4(Gains)
  Selector7/1 -> Scale gains/1
  Scale gains/1 -> Bank Angle Hold/5(Gains)
  Turn to yaw/1 -> Mux/2, Turn Rate Hold/2(Cmd)
  Selector8/1 -> Turn Rate Hold/1(Input)
  Turn to bank/1 -> Mux/1, Bank Angle Hold/3(Cmd)  "roll angle cmd"
  Selector5/1 -> Bank Angle Hold/2(Roll Angle)  "roll angle"
  Selector4/1 -> Bank Angle Hold/1(Roll Rate)
  Selector3/1 -> Turn to yaw/2
  Selector2/1 -> Turn to bank/2
  Selector1/1 -> Turn to yaw/1, Turn to bank/1
  Mux1/1 -> Display1/1, Scope8/1

== system AttitudeComplementary2/Autopilot/Yaw Control Vector Inputs ==
  note: Yaw integral
      | must be zero
  Sensors : Inport  PortDimensions=SizeSensors
  Estimates : Inport  Port=2  PortDimensions=SizeEstim
  Settings : Inport  Port=3  PortDimensions=SizeSet
  Commands : Inport  Port=4  PortDimensions=SizeCmd
  States : Inport  Port=5  PortDimensions=SizeStates
  Gains : Inport  Port=6  PortDimensions=SizeGains
  Limits : Inport  Port=7  PortDimensions=SizeLimits
  Derived : Inport  Port=8  PortDimensions=SizeDrv
  Demux : Demux  Outputs=3
  Initial condition : Constant  Value=0.0
  Mux : Mux  Inputs=3
  SaturationEx : piccolo_library/Nonlinear/SaturationEx  SystemSampleTime=-1
  Scale gains : Product  SaturateOnIntegerOverflow=on  InputSameDT=on
  Scope : Scope  NumInputPorts=3
      settings: YMin=-1~-0.015~-0.015  YMax=1~0.015~0.015  SaveName=ScopeData22
  Selector1 : Selector  IndexOptions=Index vector (dialog)  Indices=IdxSensorsYawRate  OutputSizes=1  InputPortWidth=SizeSensors
  Selector17 : Selector  IndexOptions=Index vector (dialog)  Indices=[IdxStatesGlobal IdxStatesMode IdxStatesManual]  OutputSizes=1  InputPortWidth=SizeStates
  Selector2 : Selector  IndexOptions=Index vector (dialog)  Indices=IdxDrvTurnRateCmd  OutputSizes=1  InputPortWidth=SizeDrv
  Selector3 : Selector  IndexOptions=Index vector (dialog)  Indices=IdxStatesYaw  OutputSizes=1  InputPortWidth=SizeStates
  Selector4 : Selector  IndexOptions=Index vector (dialog)  Indices=[IdxGainsYawP IdxGainsYawI IdxGainsYawD]  OutputSizes=1  InputPortWidth=SizeGains
  Selector5 : Selector  IndexOptions=Index vector (dialog)  Indices=IdxDrvGainScaler  OutputSizes=1  InputPortWidth=SizeDrv
  Selector6 : Selector  IndexOptions=Index vector (dialog)  Indices=[IdxLimitsRudderMin IdxLimitsRudderMax]  OutputSizes=1  InputPortWidth=SizeLimits
  Selector7 : Selector  IndexOptions=Index vector (dialog)  Indices=IdxSetRudderTrim  OutputSizes=1  InputPortWidth=SizeSet
  Selector8 : Selector  IndexOptions=Index vector (dialog)  Indices=IdxDrvTAS  OutputSizes=1  InputPortWidth=SizeDrv
  Sum : Sum  Inputs=-+|
  Sum1 : Sum  SaturateOnIntegerOverflow=on  InputSameDT=on
  Terminator : Terminator
  Terminator1 : Terminator
  Terminator2 : Terminator
  Turn to yaw : piccolo_library/Flight Mechanics/Turn to yaw  SystemSampleTime=-1
  Yaw Damper : piccolo_library/Controllers/PID Controller  SystemSampleTime=-1  tsamp=tsamp  tdelay=0.25
  Yaw Damper switch : piccolo_library/Logic/Yaw Damper switch  SystemSampleTime=-1
  Actuator : Outport  OutDataType=fixdt(1,16,0)  OutScaling=[]
  wires:
  Mux/1 -> Yaw Damper/4
  Demux/3 -> Mux/3
  Demux/1 -> Mux/1
  Demux/2 -> Terminator2/1
  Scale gains/1 -> Demux/1
  Commands/1 -> Terminator1/1
  Estimates/1 -> Terminator/1
  Selector1/1 -> Yaw Damper/1, Scope/2, Sum/1
  Turn to yaw/1 -> Yaw Damper/2, Scope/1, Sum/2
  Selector8/1 -> Turn to yaw/2
  Selector2/1 -> Turn to yaw/1
  Yaw Damper switch/1 -> Yaw Damper/3
  Selector3/1 -> Yaw Damper switch/2
  Selector17/1 -> Yaw Damper switch/1
  Initial condition/1 -> Mux/2, Yaw Damper/6
  Limits/1 -> Selector6/1
  Settings/1 -> Selector7/1
  Derived/1 -> Selector5/1, Selector8/1, Selector2/1
  Gains/1 -> Selector4/1
  States/1 -> Selector3/1, Selector17/1
  Sensors/1 -> Selector1/1
  Selector4/1 -> Scale gains/1
  Selector5/1 -> Scale gains/2
  Selector6/1 -> Yaw Damper/5, SaturationEx/2
  SaturationEx/1 -> Actuator/1
  Yaw Damper/1 -> Sum1/1
  Selector7/1 -> Sum1/2
  Sum1/1 -> SaturationEx/1
  Sum/1 -> Scope/3

== system AttitudeComplementary2/Get GPS in LTP/Geod2LTP2 ==
  "Height, Lat, Lon Initials from GPS" : Inport
  "Lat, deg(GPS)" : Inport  Port=2
  "Lon, deg(GPS)" : Inport  Port=3
  Hight,m(GPS) : Inport  Port=4
  Demux : Demux  Outputs=3
  ECEF2LTP (UEN) : Subsystem
      mask Display: plot(0,0,100,100,[45,40,35,40,40],[85,95,85,95,40],[85,95,85,95,40],[35,40,45,40,40],[60,40,10,20,10,14],[70,40,10,13,10,20],[56,45],[70,70],[60,60],[50,60],[60,60],[30,40],[50,60],[20,20],[30,40],[20,20],[45,55],[35,25],[75,65],[35,25])
  Geod2ECEF : Subsystem  mask{Re=6378137, Rp=6356752.3142}
      mask prompts: Re "Enter equatorial radius, m"; Rp "Enter polar radius,m"
  Geod2ECEF1 : Subsystem  mask{Re=6378137, Rp=6356752.3142}
      mask prompts: Re "Enter equatorial radius, m"; Rp "Enter polar radius,m"
  Mux : Mux  Inputs=3
  Mux1 : Mux  Inputs=2
  Mux2 : Mux  Inputs=3
  Reshape : Reshape  OutputDimensionality=Column vector (2-D)
  Sum1 : Sum  Inputs=|+-  SaturateOnIntegerOverflow=on
  UEN 2 NEU : Gain  Gain=[0 0 1;0 1 0;1 0 0]  Multiplication=Matrix(K*u)  SaturateOnIntegerOverflow=on
  "NEU, m" : Outport
  wires:
  UEN 2 NEU/1 -> "NEU, m"/1
  Geod2ECEF/3("Ze, m ") -> Mux/3
  Geod2ECEF/1("Xe, m ") -> Mux/1
  Geod2ECEF/2("Ye, m ") -> Mux/2
  "Lat, deg(GPS)"/1 -> Geod2ECEF/2("lat, deg")
  "Lon, deg(GPS)"/1 -> Geod2ECEF/3(lon,deg)
  Mux1/1 -> ECEF2LTP (UEN)/2("Long, Lat")
  Geod2ECEF1/3("Ze, m ") -> Mux2/3
  Geod2ECEF1/1("Xe, m ") -> Mux2/1
  Geod2ECEF1/2("Ye, m ") -> Mux2/2
  Mux2/1 -> Sum1/2  "R_in"
  Demux/1 -> Geod2ECEF1/1("height, m")
  Demux/2 -> Mux1/2, Geod2ECEF1/2("lat, deg")
  Demux/3 -> Mux1/1, Geod2ECEF1/3(lon,deg)
  ECEF2LTP (UEN)/1(Out) -> Reshape/1  "Moving Side"
  Hight,m(GPS)/1 -> Geod2ECEF/1("height, m")
  "Height, Lat, Lon Initials from GPS"/1 -> Demux/1
  Mux/1 -> Sum1/1  "r_mov"
  Sum1/1 -> ECEF2LTP (UEN)/1(ECEF coordinates)
  Reshape/1 -> UEN 2 NEU/1

== system AttitudeComplementary2/Get GPS in LTP/Sim Latency ==
  Fast Data : Inport
  Counter Free-Running1 : simulink/Sources/Counter Free-Running  SystemSampleTime=-1  NumBits=1  tsamp=1
  Rate Transition2 : RateTransition  OutPortSampleTime=SampleT
  Sample and Hold : dspsigops/Sample and Hold  SystemSampleTime=-1  trig=Either edge  initCond=0  latchinput=off
  1Hz Data : Outport
  wires:
  Sample and Hold/1 -> 1Hz Data/1
  Fast Data/1 -> Sample and Hold/1
  Rate Transition2/1 -> Sample and Hold/Trigger
  Counter Free-Running1/1 -> Rate Transition2/1

== system AttitudeComplementary2/Get GPS in LTP/Sim Latency3 ==
  Fast Data : Inport
  Counter Free-Running1 : simulink/Sources/Counter Free-Running  SystemSampleTime=-1  NumBits=1  tsamp=1
  Rate Transition2 : RateTransition  OutPortSampleTime=SampleT
  Sample and Hold : dspsigops/Sample and Hold  SystemSampleTime=-1  trig=Either edge  initCond=0  latchinput=off
  1Hz Data : Outport
  wires:
  Counter Free-Running1/1 -> Rate Transition2/1
  Rate Transition2/1 -> Sample and Hold/Trigger
  Fast Data/1 -> Sample and Hold/1
  Sample and Hold/1 -> 1Hz Data/1

== system AttitudeComplementary2/Get GPS in LTP/Sim Latency4 ==
  Fast Data : Inport
  Counter Free-Running1 : simulink/Sources/Counter Free-Running  SystemSampleTime=-1  NumBits=1  tsamp=1
  Rate Transition2 : RateTransition  OutPortSampleTime=SampleT
  Sample and Hold : dspsigops/Sample and Hold  SystemSampleTime=-1  trig=Either edge  initCond=0  latchinput=off
  1Hz Data : Outport
  wires:
  Sample and Hold/1 -> 1Hz Data/1
  Fast Data/1 -> Sample and Hold/1
  Rate Transition2/1 -> Sample and Hold/Trigger
  Counter Free-Running1/1 -> Rate Transition2/1

== system AttitudeComplementary2/Get GPS in LTP/Sim Latency5 ==
  Fast Data : Inport
  Counter Free-Running1 : simulink/Sources/Counter Free-Running  SystemSampleTime=-1  NumBits=1  tsamp=1
  Rate Transition2 : RateTransition  OutPortSampleTime=SampleT
  Sample and Hold : dspsigops/Sample and Hold  SystemSampleTime=-1  trig=Either edge  initCond=0  latchinput=off
  1Hz Data : Outport
  wires:
  Counter Free-Running1/1 -> Rate Transition2/1
  Rate Transition2/1 -> Sample and Hold/Trigger
  Fast Data/1 -> Sample and Hold/1
  Sample and Hold/1 -> 1Hz Data/1

== system AttitudeComplementary2/Get GPS in LTP/Sim Latency6 ==
  Fast Data : Inport
  Counter Free-Running1 : simulink/Sources/Counter Free-Running  SystemSampleTime=-1  NumBits=1  tsamp=1
  Rate Transition2 : RateTransition  OutPortSampleTime=SampleT
  Sample and Hold : dspsigops/Sample and Hold  SystemSampleTime=-1  trig=Either edge  initCond=0  latchinput=off
  1Hz Data : Outport
  wires:
  Sample and Hold/1 -> 1Hz Data/1
  Fast Data/1 -> Sample and Hold/1
  Rate Transition2/1 -> Sample and Hold/Trigger
  Counter Free-Running1/1 -> Rate Transition2/1
